simulink model "Practica1b"  (R2020b)
settings: Solver=VariableStepAuto  StartTime=0.0  StopTime=10.0  RelTol=1e-3
undefined symbols (not defined in the file or in its folder): DiscIntNeverNeededParam, K, R
libraries: pid_lib x1, simulink x1
settings Model: Creator=Danie  LastModifiedBy=Danie

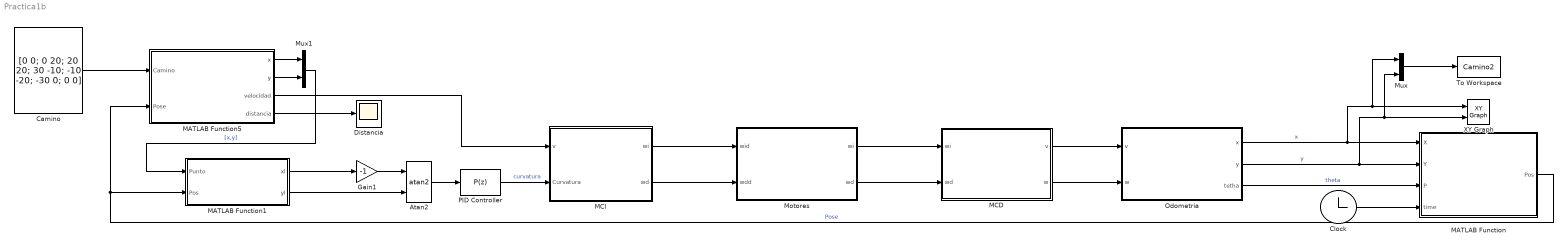
== system Practica1b ==
  Atan2 : Trigonometry  Operator=atan2
  Camino : Constant  Value=[0 0; 0 20; 20 20; 30 -10; -10 -20; -30 0; 0 0]
  Clock : Clock
      settings: Decimation=150
  Distancia : Scope
  Gain1 : Gain  Gain=-1
  MATLAB Function : MATLAB Function  TreatAsAtomicUnit=on
  MATLAB Function1 : MATLAB Function  TreatAsAtomicUnit=on
  MATLAB Function5 : MATLAB Function  TreatAsAtomicUnit=on
  MCD : Subsystem
  MCI : Subsystem
  Motores : Subsystem  mask{kwi=1, kwd=1, twi=0.12, twd=0.12}
  Mux : Mux  Inputs=2
  Mux1 : Mux  Inputs=2
  Odometria : Subsystem
  PID Controller : pid_lib/PID Controller  Controller=P  Form=Parallel  TimeDomain=Discrete-time  UseExternalTs=off  SampleTime=-1  IntegratorMethod=Forward Euler  FilterMethod=Forward Euler  ControllerParametersSource=internal  P=5.26790729973159  I=1  D=0  UseFilter=on  N=100  TunerSelectOption=Transfer Function Based (PID Tuner App)  InitialConditionSource=internal  InitialConditionForIntegrator=0  InitialConditionForFilter=0  DifferentiatorICPrevScaledInput=0  ExternalReset=none  TrackingMode=off  Kt=1  LimitOutput=off  SatLimitsSource=internal  UpperSaturationLimit=inf  LowerSaturationLimit=-inf  LinearizeAsGain=on  AntiWindupMode=none  Kb=1  POutMin=[]  POutMax=[]  IOutMin=[]  IOutMax=[]  DOutMin=[]  DOutMax=[]  NOutMin=[]  NOutMax=[]  SumOutMin=[]  SumOutMax=[]  SaturationOutMin=[]  SaturationOutMax=[]  PParamMin=[]  PParamMax=[]  IParamMin=[]  IParamMax=[]  DParamMin=[]  DParamMax=[]  NParamMin=[]  NParamMax=[]  KbParamMin=[]  KbParamMax=[]  KtParamMin=[]  KtParamMax=[]  KbOutMin=[]  KbOutMax=[]  KtOutMin=[]  KtOutMax=[]  IntegratorOutMin=[]  IntegratorOutMax=[]  FilterOutMin=[]  FilterOutMax=[]  SumI1OutMin=[]  SumI1OutMax=[]  SumI2OutMin=[]  SumI2OutMax=[]  SumI3OutMin=[]  SumI3OutMax=[]  SumI4OutMin=[]  SumI4OutMax=[]  SumDOutMin=[]  SumDOutMax=[]  DifferentiatorOutMin=[]  DifferentiatorOutMax=[]  FilterDiffOutCoefMin=[]  FilterDiffOutCoefMax=[]  ReciprocalOutMin=[]  ReciprocalOutMax=[]  SumDenOutMin=[]  SumDenOutMax=[]  SumNumOutMin=[]  SumNumOutMax=[]  DivideOutMin=[]  DivideOutMax=[]  UdiffTsProdOutMin=[]  UdiffTsProdOutMax=[]  NTsProdOutMin=[]  NTsProdOutMax=[]  UintegralTsProdOutMin=[]  UintegralTsProdOutMax=[]  UngainTsProdOutMin=[]  UngainTsProdOutMax=[]  IntegratorContinuousStateAttributes=''  IntegratorStateMustResolveToSignalObject=off  IntegratorRTWStateStorageClass=Auto  FilterContinuousStateAttributes=''  FilterStateMustResolveToSignalObject=off  FilterRTWStateStorageClass=Auto  ParallelPVariant=InternalParameters  IdealPVariant=Disabled  IVariant=Disabled  DVariant=Disabled  IntegratorVariant=Disabled  SatVariant=Disabled  AWVariant=Disabled  PCopyVariant=Disabled  TRVariant=Disabled  FdbkBlocksVariant=Forward  IdealPFdbkVariant=Disabled  SatFdbkVariant=Disabled  DerivativeFilterVariant=Disabled  NVariant=Disabled  NCopyVariant=Disabled_SignalSpec  FilterICVariant=Disabled  IntegratorICVariant=Disabled  ExternalResetVariant=Disabled  TRSumVariant=Passthrough  SumFdbkVariant=Disabled  SumVariant=Passthrough_P  TsampFilterVariant=InternalTs  TsampNgainVariant=Passthrough  TsampIntegralVariant=Disabled_SignalSpec  ExternalSaturationOutDataTypeStr=Inherit: Same as second input
  To Workspace : ToWorkspace  VariableName=Camino2  SaveFormat=Structure  SampleTime=-1
  XY Graph : simulink/Sinks/XY Graph  xmin=-50  xmax=50  ymin=-50  ymax=50  st=-1
  wires:
  MCD/1(v) -> Odometria/1(v)
  Gain1/1 -> Atan2/1
  Atan2/1 -> PID Controller/1
  MATLAB Function5/4(distancia) -> Distancia/1
  MATLAB Function5/2(y) -> Mux1/2
  Odometria/1(x) -> Mux/1, XY Graph/1, MATLAB Function/1(X)  "x"
  MATLAB Function1/2(yl) -> Atan2/2
  MATLAB Function5/1(x) -> Mux1/1
  MATLAB Function5/3(velocidad) -> MCI/1(v)
  MCI/2(wd) -> Motores/2(wdd)
  MATLAB Function/1(Pos) -> MATLAB Function1/2(Pos), MATLAB Function5/2(Pose)  "Pose"
  Motores/1(wi) -> MCD/1(wi)
  Odometria/3(tetha) -> MATLAB Function/3(P)  "theta"
  Mux1/1 -> MATLAB Function1/1(Punto)  "[x,y]"
  MATLAB Function1/1(xl) -> Gain1/1
  MCI/1(wi) -> Motores/1(wid)
  Clock/1 -> MATLAB Function/4(time)
  Motores/2(wd) -> MCD/2(wd)
  Camino/1 -> MATLAB Function5/1(Camino)
  MCD/2(w) -> Odometria/2(w)
  Mux/1 -> To Workspace/1
  Odometria/2(y) -> Mux/2, XY Graph/2, MATLAB Function/2(Y)  "y"
  PID Controller/1 -> MCI/2(Curvatura)  "curvatura"

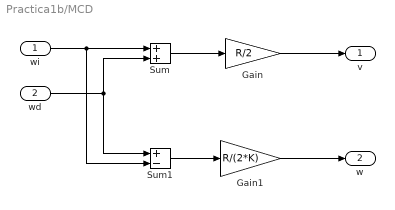
== system Practica1b/MCD ==
  wi : Inport
  wd : Inport  Port=2
  Gain : Gain  Gain=R/2
  Gain1 : Gain  Gain=R/(2*K)
  Sum : Sum
  Sum1 : Sum  Inputs=+-
  v : Outport  VectorParamsAs1DForOutWhenUnconnected=off
  w : Outport  Port=2  VectorParamsAs1DForOutWhenUnconnected=off
  wires:
  Gain/1 -> v/1
  wi/1 -> Sum1/2, Sum/1
  wd/1 -> Sum1/1, Sum/2
  Sum/1 -> Gain/1
  Gain1/1 -> w/1
  Sum1/1 -> Gain1/1

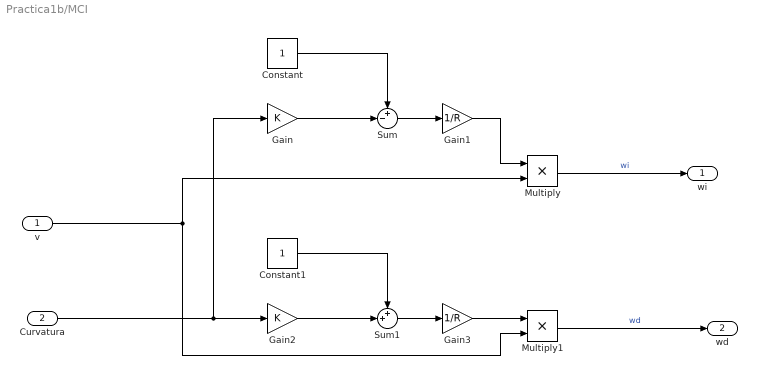
== system Practica1b/MCI ==
  v : Inport
  Curvatura : Inport  Port=2
  Constant : Constant
  Constant1 : Constant
  Gain : Gain  Gain=K
  Gain1 : Gain  Gain=1/R
  Gain2 : Gain  Gain=K
  Gain3 : Gain  Gain=1/R
  Multiply : Product
  Multiply1 : Product
  Sum : Sum  Inputs=+-|
  Sum1 : Sum  Inputs=++|
  wi : Outport  VectorParamsAs1DForOutWhenUnconnected=off
  wd : Outport  Port=2  VectorParamsAs1DForOutWhenUnconnected=off
  wires:
  Gain3/1 -> Multiply1/1
  v/1 -> Multiply/2, Multiply1/2
  Gain2/1 -> Sum1/2
  Gain1/1 -> Multiply/1
  Gain/1 -> Sum/2
  Constant1/1 -> Sum1/1
  Curvatura/1 -> Gain/1, Gain2/1
  Sum1/1 -> Gain3/1
  Sum/1 -> Gain1/1
  Constant/1 -> Sum/1
  Multiply1/1 -> wd/1  "wd"
  Multiply/1 -> wi/1  "wi"

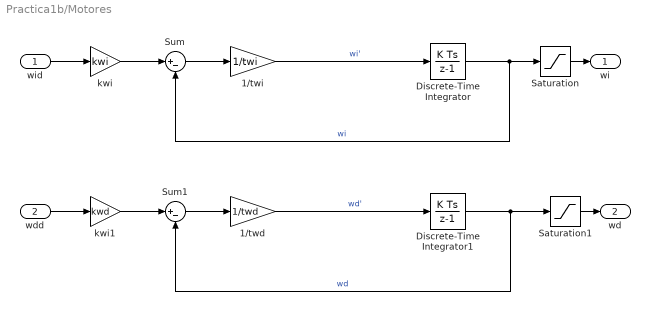
== system Practica1b/Motores ==
  wid : Inport
  wdd : Inport  Port=2
  1/twd : Gain  Gain=1/twd
  1/twi : Gain  Gain=1/twi
  Discrete-Time Integrator : DiscreteIntegrator  SampleTime=0.025  ICPrevOutput=DiscIntNeverNeededParam  ICPrevScaledInput=DiscIntNeverNeededParam
  Discrete-Time Integrator1 : DiscreteIntegrator  SampleTime=0.025  ICPrevOutput=DiscIntNeverNeededParam  ICPrevScaledInput=DiscIntNeverNeededParam
  Saturation : Saturate  UpperLimit=15  LowerLimit=-15
  Saturation1 : Saturate  UpperLimit=15  LowerLimit=-15
  Sum : Sum  Inputs=|+-
  Sum1 : Sum  Inputs=|+-
  kwi : Gain  Gain=kwi
  kwi1 : Gain  Gain=kwd
  wi : Outport  VectorParamsAs1DForOutWhenUnconnected=off
  wd : Outport  Port=2  VectorParamsAs1DForOutWhenUnconnected=off
  wires:
  kwi/1 -> Sum/1
  Discrete-Time Integrator/1 -> Sum/2, Saturation/1  "wi"
  Sum/1 -> 1/twi/1
  Saturation/1 -> wi/1
  1/twi/1 -> Discrete-Time Integrator/1  "wi'"
  Discrete-Time Integrator1/1 -> Sum1/2, Saturation1/1  "wd"
  wid/1 -> kwi/1
  1/twd/1 -> Discrete-Time Integrator1/1  "wd'"
  kwi1/1 -> Sum1/1
  Sum1/1 -> 1/twd/1
  Saturation1/1 -> wd/1
  wdd/1 -> kwi1/1

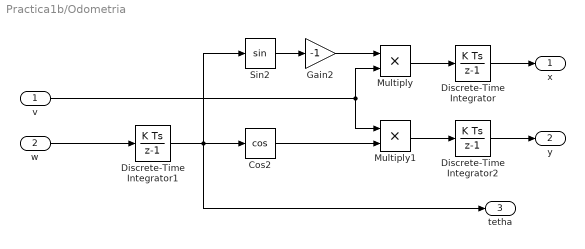
== system Practica1b/Odometria ==
  v : Inport
  w : Inport  Port=2
  Cos2 : Trigonometry  Operator=cos
  Discrete-Time Integrator : DiscreteIntegrator  SampleTime=-1  ICPrevOutput=DiscIntNeverNeededParam  ICPrevScaledInput=DiscIntNeverNeededParam
  Discrete-Time Integrator1 : DiscreteIntegrator  SampleTime=-1  ICPrevOutput=DiscIntNeverNeededParam  ICPrevScaledInput=DiscIntNeverNeededParam
  Discrete-Time Integrator2 : DiscreteIntegrator  SampleTime=-1  ICPrevOutput=DiscIntNeverNeededParam  ICPrevScaledInput=DiscIntNeverNeededParam
  Gain2 : Gain  Gain=-1
  Multiply : Product
  Multiply1 : Product
  Sin2 : Trigonometry
  x : Outport  VectorParamsAs1DForOutWhenUnconnected=off
  y : Outport  Port=2  VectorParamsAs1DForOutWhenUnconnected=off
  tetha : Outport  Port=3  VectorParamsAs1DForOutWhenUnconnected=off
  wires:
  Multiply1/1 -> Discrete-Time Integrator2/1
  Discrete-Time Integrator1/1 -> Cos2/1, Sin2/1, tetha/1
  w/1 -> Discrete-Time Integrator1/1
  v/1 -> Multiply1/1, Multiply/2
  Multiply/1 -> Discrete-Time Integrator/1
  Sin2/1 -> Gain2/1
  Cos2/1 -> Multiply1/2
  Gain2/1 -> Multiply/1
  Discrete-Time Integrator/1 -> x/1
  Discrete-Time Integrator2/1 -> y/1

== matlab function Practica1b/MATLAB Function1 ==
  data: Punto input; xl output; Pos input; yl output
function [xl,yl] = locales(Punto,Pos)

x0=Pos(1);
y0=Pos(2);
tita=Pos(3);

x=Punto(1);
y=Punto(2);

xl=(x-x0)*cos(tita)+(y-y0)*sin(tita);
yl=-(x-x0)*sin(tita)+(y-y0)*cos(tita);

== matlab function Practica1b/MATLAB Function ==
  data: X input; Pos output; Y input; P input; time input
function Pos = DGPS(X, Y, P,time)

Pos=[0;0;0];
pos= [X; Y; P]+sqrtm([0.4 -0.014 0; -0.014 0.5 0;0 0 0.1])*randn(3, 1);
persistent xp yp angulop;
if isempty(xp)||isempty(yp)||isempty(angulop)
    xp=0;
    yp=0;
    angulop=0;
end
if mod(time,0.3)==0
    xp=real(pos(1));
    yp=real(pos(2));
    angulop=real(pos(3));
end
Pos(1)=xp;
Pos(2)=yp;
Pos(3)=angulop;
end

== matlab function Practica1b/MATLAB Function5 ==
  data: x output; Camino input; y output; velocidad output; Pose input; distancia output
function [x,y,velocidad,distancia]= Seleccion_Camino(Camino,Pose)

persistent i vel;

if isempty(i)||isempty(vel)
    i=1;
    vel=1.2;
end

[l,r]=size(Camino);

dx=Camino(i,1)-Pose(1);
dy=Camino(i,2)-Pose(2);
d=[dx,dy];
distancia=norm(d);

if distancia<1          
    i=i+1;    
    vel=1.2; 
end



if i>l
    i=l-1;     
    vel=0;     
end

x=Camino(i,1);
y=Camino(i,2);
velocidad=vel;
